simulink model "PID_20141024"  (Simulink 7.4)
settings: Solver=ode1  StartTime=0.0  StopTime=10  FixedStep=0.005  RelTol=1e-3
settings Model: Creator=jinsx  LastModifiedBy=jinsx

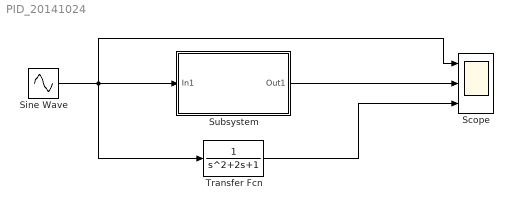
== system PID_20141024 ==
  Scope : Scope  NumInputPorts=3
      settings: YMin=0~-5~-5  YMax=20~5~5
  Sine Wave : Sin  Amplitude=1  Bias=0  Frequency=1  Phase=0  Samples=10  SampleTime=0  Offset=0
  Subsystem : Subsystem
  Transfer Fcn : TransferFcn
  wires:
  Sine Wave/1 -> Subsystem/1(In1), Scope/1, Transfer Fcn/1
  Transfer Fcn/1 -> Scope/3
  Subsystem/1(Out1) -> Scope/2

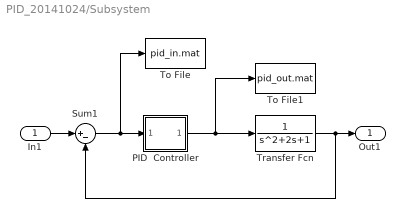
== system PID_20141024/Subsystem ==
  In1 : Inport
  PID  Controller : Subsystem  mask(PID Controller){P=0, I=0, D=5}
      mask prompts: P "Propotioan"; I "Integral"; D "Differetial"
      mask help:
      | Enter expressions for proportional, integral, and derivative terms.
      | P+I/s+Ds
      mask Help: This block implements a PID controller where parameters are entered for the Proportional, Integral and Derivative terms. Unmask this block to see how it works. The derivative term is implemented using a true derivative block.
      mask Display: disp('PID')
  Sum1 : Sum  Inputs=|+-  OutDataType=fixdt(1, 16)  OutScaling=2^0
  To File : ToFile  Filename=pid_in.mat
  To File1 : ToFile  Filename=pid_out.mat
  Transfer Fcn : TransferFcn
  Out1 : Outport
  wires:
  Transfer Fcn/1 -> Sum1/2, Out1/1
  PID  Controller/1(Out_1) -> To File1/1, Transfer Fcn/1
  Sum1/1 -> To File/1, PID  Controller/1(In_1)
  In1/1 -> Sum1/1

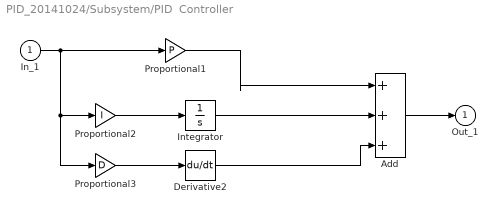
== system PID_20141024/Subsystem/PID  Controller ==
  In_1 : Inport
  Add : Sum  Inputs=+++  OutDataType=fixdt(1, 16)  OutScaling=2^-10
  Derivative2 : Derivative
  Integrator : Integrator
  Proportional1 : Gain  Gain=P  SaturateOnIntegerOverflow=on  OutDataTypeStr=Inherit: Same as input  ParamDataTypeStr=Inherit: Same as input
  Proportional2 : Gain  Gain=I  SaturateOnIntegerOverflow=on  OutDataTypeStr=Inherit: Same as input  ParamDataTypeStr=Inherit: Same as input
  Proportional3 : Gain  Gain=D  SaturateOnIntegerOverflow=on  OutDataTypeStr=Inherit: Same as input  ParamDataTypeStr=Inherit: Same as input
  Out_1 : Outport  InitialOutput=0
  wires:
  In_1/1 -> Proportional1/1, Proportional2/1, Proportional3/1
  Integrator/1 -> Add/2
  Proportional2/1 -> Integrator/1
  Derivative2/1 -> Add/3
  Proportional3/1 -> Derivative2/1
  Add/1 -> Out_1/1
  Proportional1/1 -> Add/1
